simulink model "Demo_MinSegMotor"  (R2015a)
settings: Solver=FixedStepDiscrete  SolverMode=SingleTasking  StartTime=0.0  StopTime=inf  FixedStep=.03  RelTol=1e-3
PostLoadFcn:
  | try,
  | codertarget.arduinobase.registry.setBaudRate(gcs,115200)
  | disp('baud rate set to 115200 for external mode hardware serial')
  | baudrate='set_to_115200'
  | catch
  | disp('baud rate setting not needed in this version')
  | end
libraries: MinSegLibrary_M2V5 x4, arduinolib x3, RASPlib x2
settings Model: SimulationMode=external  ExtModeTrigDuration=2  Creator=Alec  LastModifiedBy=hurstj
settings OptimizationCC: ExpressionDepthLimit=2147483647  OptimizeModelRefInitCode=on  LifeSpan=1
settings DebuggingCC: UnderspecifiedInitializationDetection=Classic  MergeDetectMultiDrivingBlocksExec=none  StateNameClashWarn=warning
settings HardwareCC: ProdBitPerInt=16  ProdBitPerPointer=8  ProdIntDivRoundTo=Zero  ProdEndianess=LittleEndian  ProdWordSize=8  ProdHWDeviceType=Atmel->AVR
settings RTWCC: SystemTargetFile=realtime.tlc  GenerateMakefile=off  TemplateMakefile=realtime.tmf  Description=Real-Time Toolbox  RTWVerbose=off
settings CodeAppCC: CustomSymbolStrType=$N$R$M  InternalIdentifier=Classic
settings ERTTargetCC: CombineOutputUpdateFcns=off  ExtMode=on  ExtModeTransport=3  ExtModeMexArgs=0 89 115200  ERTSrcFileBannerTemplate=realtime_code_template.cgt  ERTHdrFileBannerTemplate=realtime_code_template.cgt  ERTDataSrcFileTemplate=realtime_code_template.cgt  ERTDataHdrFileTemplate=realtime_code_template.cgt  ERTCustomFileTemplate=realtime_file_process.tlc

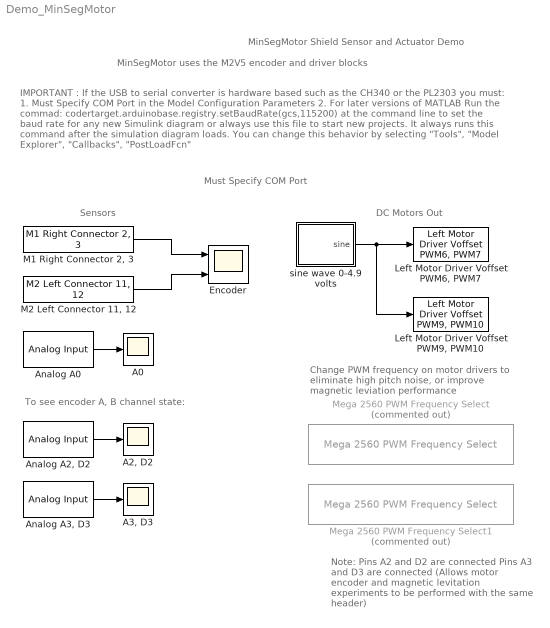
== system Demo_MinSegMotor ==
  note: MinSegMotor uses the M2V5 encoder and driver blocks
  note: To see encoder A, B channel state:
  note: IMPORTANT : If the USB to serial converter is hardware based such as the CH340 or the PL2303 you must:
      | 1. Must Specify COM Port in the Model Configuration Parameters
      | 2. For later versions of MATLAB Run the commad: codertarget.arduinobase.registry.setBaudRate(gcs,115200)
      | at the command line to set the baud rate for any new Simulink diagram or always use this file to start new projects.
      | It always runs this command after the simulation diagram loads.
      | You can change this behavior by selecting "Tools", "Model Explorer", "Callbacks", "PostLoadFcn"
  note: Must Specify COM Port
  note: Note: Pins  A2 and D2 are connected
      |          Pins  A3 and D3 are connected
      | (Allows  motor encoder and magnetic
      | levitation experiments to be performed
      | with the same header)
  note: DC Motors Out
  note: Sensors
  note: MinSegMotor Shield Sensor and Actuator Demo
  note: Change PWM frequency on motor drivers
      | to eliminate high pitch noise, or improve
      | magnetic leviation performance
  A0 : Scope
      settings: TimeRange=30  YMin=0  YMax=1100  SaveName=ScopeData2  ScrollMode=on
  "A2, D2" : Scope
      settings: TimeRange=30  SaveName=ScopeData5
  "A3, D3" : Scope
      settings: TimeRange=30  SaveName=ScopeData4
  Analog A0 : arduinolib/Analog Input  pinNumber=0  sampleTime=-1  blockPlatform=arduino
  "Analog A2, D2" : arduinolib/Analog Input  pinNumber=2  sampleTime=-1  blockPlatform=arduino
  "Analog A3, D3" : arduinolib/Analog Input  pinNumber=3  sampleTime=-1  blockPlatform=arduino
  Encoder : Scope  NumInputPorts=2
      settings: TimeRange=30  YMin=-4000~-4000  YMax=4000~4000  ScrollMode=on
  "Left Motor Driver Voffset PWM6, PWM7" : MinSegLibrary_M2V5/Left Motor Driver Voffset PWM6, PWM7  Vsupply=4.9  Voffset=0
  "Left Motor Driver Voffset PWM9, PWM10" : MinSegLibrary_M2V5/Left Motor Driver Voffset PWM9, PWM10  Vsupply=4.9  Voffset=0
  "M1 Right Connector 2, 3" : MinSegLibrary_M2V5/M1 Right Connector 2, 3  Encoder=0  PinA=2  PinB=3
  "M2 Left Connector 11, 12" : MinSegLibrary_M2V5/M2 Left Connector 11, 12  Encoder=4  PinA=11  PinB=12
  Mega 2560 PWM Frequency Select : RASPlib/Mega 2560 PWM Frequency Select  Commented=on  Frequency=32KHz  Timer=4 - pins 6, 7, 8
  Mega 2560 PWM Frequency Select1 : RASPlib/Mega 2560 PWM Frequency Select  Commented=on  Frequency=32KHz  Timer=2 - pins 9, 10
  sine wave 0-4.9 volts : Subsystem
  wires:
  sine wave 0-4.9 volts/1(sine) -> "Left Motor Driver Voffset PWM9, PWM10"/1, "Left Motor Driver Voffset PWM6, PWM7"/1
  "M1 Right Connector 2, 3"/1 -> Encoder/1
  "M2 Left Connector 11, 12"/1 -> Encoder/2
  Analog A0/1 -> A0/1
  "Analog A2, D2"/1 -> "A2, D2"/1
  "Analog A3, D3"/1 -> "A3, D3"/1

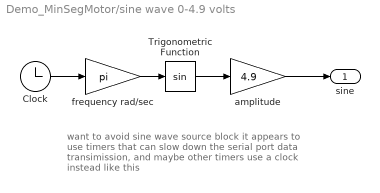
== system Demo_MinSegMotor/sine wave 0-4.9 volts ==
  note: want to avoid sine wave source block
      | it appears to use timers that can slow down the
      | serial port data transimission, and maybe
      | other timers
      |
      | use a clock instead like this
  Clock : Clock
  Trigonometric Function : Trigonometry
  amplitude : Gain  Gain=4.9
  frequency rad/sec : Gain  Gain=pi
  sine : Outport
  wires:
  Clock/1 -> frequency rad/sec/1
  Trigonometric Function/1 -> amplitude/1
  frequency rad/sec/1 -> Trigonometric Function/1
  amplitude/1 -> sine/1
